simulink model "sistema_completo_con_observador_de_estado"  (R2023b)
settings: Solver=VariableStepAuto  StartTime=0.0  StopTime=10.0  RelTol=1e-3
values from neighbouring files (symbols this model uses):
  alpha_Cu = 3.9e-3    (= 0.0039)    [controlador_foc_simulink.m]    (also in parametros_planta.m; params_subsistema_termico.m; sistema_completo_en_codigo.m)
  ba_num = Jeq_ctrl*n_pid*wn_pid    (= 0.0395694444444)    [controlador_foc_simulink.m]    (also in sistema_completo_en_codigo.m)
  beq_nom = bm + bl_nom/r^2    (= 2.19444444444e-05)    [parametros_planta.m]    (also in params_subsistema_mecanico.m; sistema_completo_en_codigo.m)
  Cts = 0.818    [parametros_planta.m]    (also in params_subsistema_termico.m)
  g = 9.80665    [controlador_foc_simulink.m]    (also in parametros_planta.m; params_subsistema_mecanico.m; sistema_completo_en_codigo.m)
  Jeq_nom = Jm + Jl_nom/r^2    (= 1.97847222222e-05)    [params_subsistema_mecanico.m]    (also in sistema_completo_en_codigo.m)
  kg_eq_nom = g*kl_nom/r    (= 0.0204305208333)    [params_subsistema_mecanico.m]    (also in sistema_completo_en_codigo.m)
  kl_nom = m*Lcm + ml_nom*Ll    (= 0.25)    [controlador_foc_simulink.m]    (also in params_subsistema_mecanico.m; sistema_completo_en_codigo.m)
  Ksa_num = Jeq_ctrl*n_pid*wn_pid^2    (= 31.6555555556)    [controlador_foc_simulink.m]    (also in sistema_completo_en_codigo.m)
  Ksia_num = Jeq_ctrl*wn_pid^3    (= 10129.7777778)    [controlador_foc_simulink.m]    (also in sistema_completo_en_codigo.m)
  L_d = 6.6e-3    (= 0.0066)    [controlador_foc_simulink.m]    (also in params_subsistema_electromagnetico.m; sistema_completo_en_codigo.m)
  L_l = 0.8e-3    (= 0.0008)    [controlador_foc_simulink.m]    (also in params_subsistema_electromagnetico.m; sistema_completo_en_codigo.m)
  L_q = 5.8e-3    (= 0.0058)    [controlador_foc_simulink.m]    (also in params_subsistema_electromagnetico.m; sistema_completo_en_codigo.m)
  lambda_m = 0.016    [controlador_foc_simulink.m]    (also in parametros_planta.m; params_subsistema_electromagnetico.m; sistema_completo_en_codigo.m)
  Pp = 3    [controlador_foc_simulink.m]    (also in parametros_planta.m; params_subsistema_electromagnetico.m; sistema_completo_en_codigo.m)
  r = 120.0    (= 120)    [controlador_foc_simulink.m]    (also in parametros_planta.m; params_subsistema_mecanico.m; sistema_completo_en_codigo.m)
  Rs_REF = 1.02    [controlador_foc_simulink.m]    (also in parametros_planta.m; params_subsistema_termico.m; sistema_completo_en_codigo.m)
  Rts_amb = 146.7    [parametros_planta.m]    (also in params_subsistema_termico.m)
  Tamb = Tamb_max    (= 40)    [parametros_planta.m]    (also in params_subsistema_termico.m; sistema_completo_en_codigo.m)
  Ts_REF = 20.0    (= 20)    [controlador_foc_simulink.m]    (also in parametros_planta.m; params_subsistema_termico.m; sistema_completo_en_codigo.m)
settings Model: Creator=Pc  LastModifiedBy=Pc

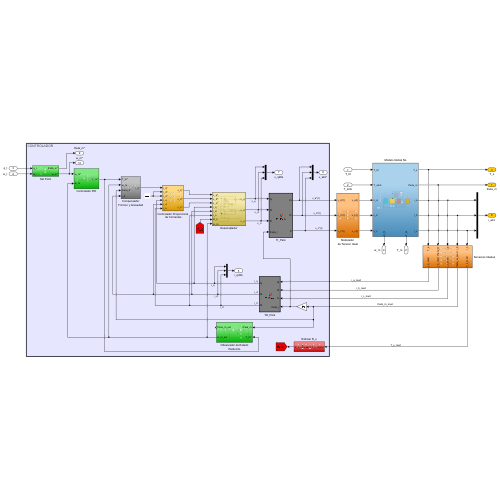
[thumbnail: Simulink's stored preview of the top-level diagram]
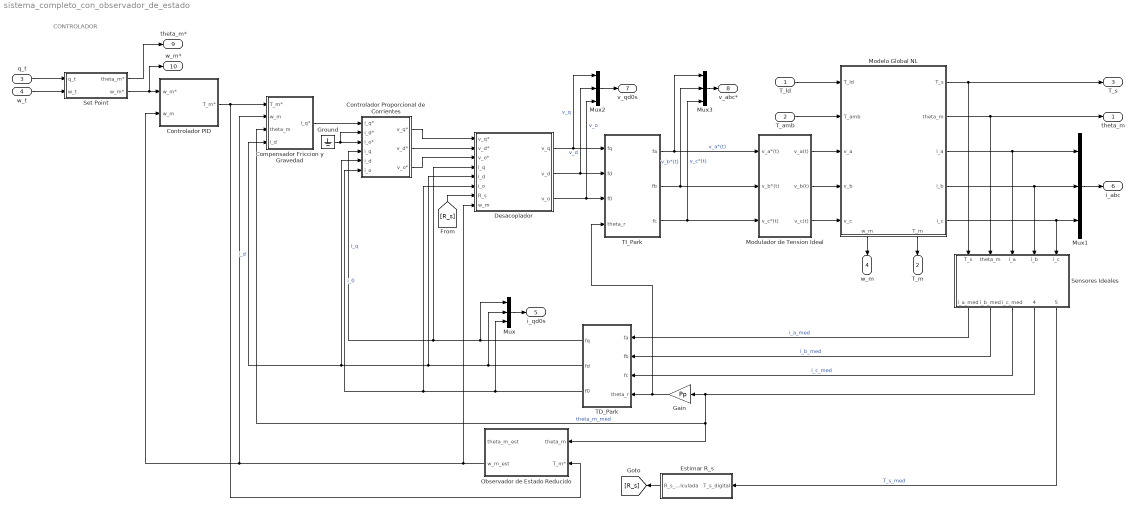
== system sistema_completo_con_observador_de_estado ==
  note: CONTROLADOR
  T_ld : Inport
  T_amb : Inport  Port=2
  q_t : Inport  Port=3
  w_t : Inport  Port=4
  Compensador Friccion y Gravedad : Subsystem
  Controlador PID : Subsystem
  Controlador Proporcional de Corrientes : Subsystem
  Desacoplador : Subsystem
  Estimar R_s : Subsystem
  Gain : Gain  Gain=Pp
  Ground : Ground
  Modelo Global NL : Subsystem
      settings: PortSchema="{\"entries\":[{\"content\":{\"sides\":[{\"content\":{\"connectorIds\":[\"In1\",\"In2\",\"In3\",\"In4\",\"In5\"]},\"type\":\"ConnectorPlacement.EquallySpacedRectSide\",\"uuid\":\"386252be-5f39-4928-a151-52e681895a84\"},{\"content\":{\"connectorIds\":[\"Out1\",\"Out2\",\"Out3\",\"Out4\",\"Out5\"],\"side\":\"RIGHT\"},\"type\":\"ConnectorPlacement.EquallySpacedRectSide\",\"uuid\":\"aee83b90-e95b-4477-b157-a5534e7c5e6c\"},{\"content\":{\"side\":\"TOP\"},\"type\":\"ConnectorPlacement.EquallySpacedRectSide\",\"uuid\":\"e739b3f7-cae1-4498-b396-d13f7405e232\"},{\"content\":{\"connectorIds\":[\"Out6\",\"Out7\"],\"side\":\"BOTTOM\"},\"type\":\"ConnectorPlacement.EquallySpacedRectSide\",\"uuid\":\"86304fed-22cd-46a2-87e5-e7bae1c5cedf\"}]},\"type\":\"ConnectorPlacement.EquallySpacedConnector\",\"uuid\":\"c0eb110b-b212-4702-a1d5-9ec3ac2ff196\"}],\"packageUris\":[\"http://schema.mathworks.com/mf0/Connector/R2020b\"],\"version\":\"1.0\"}"
  Modulador de Tension Ideal : Subsystem
  Mux{,1..3} (4 alike) : Mux  Inputs=3
  Observador de Estado Reducido : Subsystem
  Sensores Ideales : Subsystem
  Set Point : Subsystem
  TD_Park : MATLAB Function  TreatAsAtomicUnit=on
  TI_Park : MATLAB Function  TreatAsAtomicUnit=on
  theta_m : Outport
  T_m : Outport  Port=2
  T_s : Outport  Port=3
  w_m : Outport  Port=4
  i_qd0s : Outport  Port=5
  i_abc : Outport  Port=6
  v_qd0s : Outport  Port=7
  v_abc* : Outport  Port=8
  theta_m* : Outport  Port=9
  w_m* : Outport  Port=10
  wires:
  Sensores Ideales/2(i_b_med) -> TD_Park/2(fb)  "i_b_med"
  Modulador de Tension Ideal/2(v_b(t)) -> Modelo Global NL/4(v_b)
  Mux2/1 -> v_qd0s/1
  TI_Park/2(fb) -> Modulador de Tension Ideal/2(v_b*(t)), Mux3/2  "v_b*(t)"
  Desacoplador/3(v_o) -> Mux2/3, TI_Park/3(f0)  "v_o"
  Mux1/1 -> i_abc/1
  Sensores Ideales/4(theta_m_med) -> Observador de Estado Reducido/1(theta_m), Compensador Friccion y Gravedad/3(theta_m), Gain/1  "theta_m_med"
  TD_Park/2(fd) -> Compensador Friccion y Gravedad/4(i_d), Controlador Proporcional de Corrientes/5(i_d), Desacoplador/5(i_d), Mux/2  "i_d"
  Modelo Global NL/1(T_s) -> T_s/1, Sensores Ideales/1(T_s)
  Modulador de Tension Ideal/1(v_a(t)) -> Modelo Global NL/3(v_a)
  Desacoplador/1(v_q) -> Mux2/1, TI_Park/1(fq)  "v_q"
  TD_Park/1(fq) -> Desacoplador/4(i_q), Controlador Proporcional de Corrientes/4(i_q), Mux/1  "i_q"
  TI_Park/3(fc) -> Modulador de Tension Ideal/3(v_c*(t)), Mux3/3  "v_c*(t)"
  Modelo Global NL/5(i_c) -> Mux1/3, Sensores Ideales/5(i_c)
  Mux/1 -> i_qd0s/1
  Gain/1 -> TI_Park/4(theta_r), TD_Park/4(theta_r)
  Modelo Global NL/7(T_m) -> T_m/1
  Mux3/1 -> v_abc*/1
  Sensores Ideales/3(i_c_med) -> TD_Park/3(fc)  "i_c_med"
  TD_Park/3(f0) -> Controlador Proporcional de Corrientes/6(i_o), Desacoplador/6(i_o), Mux/3  "i_0"
  Sensores Ideales/1(i_a_med) -> TD_Park/1(fa)  "i_a_med"
  Modulador de Tension Ideal/3(v_c(t)) -> Modelo Global NL/5(v_c)
  Modelo Global NL/2(theta_m) -> theta_m/1, Sensores Ideales/2(theta_m)
  T_amb/1 -> Modelo Global NL/2(T_amb)
  T_ld/1 -> Modelo Global NL/1(T_ld)
  TI_Park/1(fa) -> Mux3/1, Modulador de Tension Ideal/1(v_a*(t))  "v_a*(t)"
  Modelo Global NL/3(i_a) -> Mux1/1, Sensores Ideales/3(i_a)
  Modelo Global NL/4(i_b) -> Mux1/2, Sensores Ideales/4(i_b)
  Desacoplador/2(v_d) -> Mux2/2, TI_Park/2(fd)  "v_d"
  Controlador Proporcional de Corrientes/2(v_d*) -> Desacoplador/2(v_d*)
  Controlador Proporcional de Corrientes/3(v_o*) -> Desacoplador/3(v_o*)
  Controlador Proporcional de Corrientes/1(v_q*) -> Desacoplador/1(v_q*)
  Ground/1 -> Controlador Proporcional de Corrientes/2(i_d*), Controlador Proporcional de Corrientes/3(i_o*)
  Compensador Friccion y Gravedad/1(i_q*) -> Controlador Proporcional de Corrientes/1(i_q*)
  Controlador PID/1(T_m*) -> Observador de Estado Reducido/2(T_m*), Compensador Friccion y Gravedad/1(T_m*)
  q_t/1 -> Set Point/1(q_t)
  w_t/1 -> Set Point/2(w_t)
  Set Point/2(w_m*) -> w_m*/1, Controlador PID/1(w_m*)
  Set Point/1(theta_m*) -> theta_m*/1
  Estimar R_s/1(R_s_calculada) -> [R_s]
  [R_s] -> Desacoplador/7(R_s)
  Modelo Global NL/6(w_m) -> w_m/1
  Observador de Estado Reducido/2(w_m_est) -> Controlador PID/2(w_m), Compensador Friccion y Gravedad/2(w_m), Desacoplador/8(w_m)
  Sensores Ideales/5(T_s_med) -> Estimar R_s/1(T_s_digital)  "T_s_med"

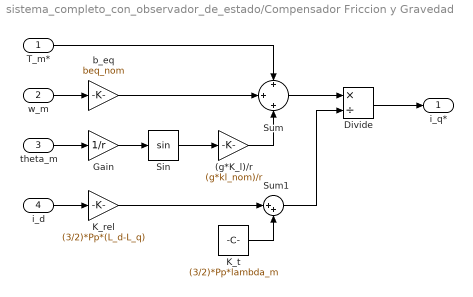
== system sistema_completo_con_observador_de_estado/Compensador Friccion y Gravedad ==
  T_m* : Inport
  w_m : Inport  Port=2
  theta_m : Inport  Port=3
  i_d : Inport  Port=4
  (g*K_l)/r : Gain  Gain=(g*kl_nom)/r
  Divide : Product  Inputs=*/
  Gain : Gain  Gain=1/r
  K_rel : Gain  Gain=(3/2)*Pp*(L_d-L_q)
  K_t : Constant  Value=(3/2)*Pp*lambda_m
  Sin : Trigonometry
  Sum : Sum  Inputs=+|+|+
  Sum1 : Sum  Inputs=|++
  b_eq : Gain  Gain=beq_nom
  i_q* : Outport
  wires:
  i_d/1 -> K_rel/1
  T_m*/1 -> Sum/1
  Sin/1 -> (g*K_l)/r/1
  K_t/1 -> Sum1/2
  (g*K_l)/r/1 -> Sum/3
  Sum1/1 -> Divide/2
  Gain/1 -> Sin/1
  b_eq/1 -> Sum/2
  K_rel/1 -> Sum1/1
  w_m/1 -> b_eq/1
  Sum/1 -> Divide/1
  Divide/1 -> i_q*/1
  theta_m/1 -> Gain/1

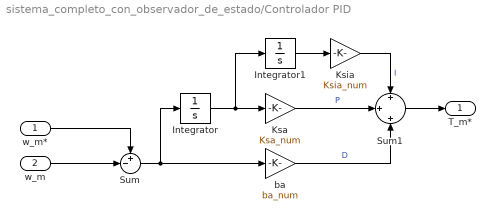
== system sistema_completo_con_observador_de_estado/Controlador PID ==
  w_m* : Inport
  w_m : Inport  Port=2
  Integrator : Integrator
  Integrator1 : Integrator
  Ksa : Gain  Gain=Ksa_num
  Ksia : Gain  Gain=Ksia_num
  Sum : Sum  Inputs=+-|
  Sum1 : Sum  Inputs=+|+|+
  ba : Gain  Gain=ba_num
  T_m* : Outport
  wires:
  Sum1/1 -> T_m*/1
  Ksa/1 -> Sum1/2  "P"
  Ksia/1 -> Sum1/1  "I"
  ba/1 -> Sum1/3  "D"
  Integrator/1 -> Integrator1/1, Ksa/1
  Integrator1/1 -> Ksia/1
  Sum/1 -> Integrator/1, ba/1
  w_m*/1 -> Sum/1
  w_m/1 -> Sum/2

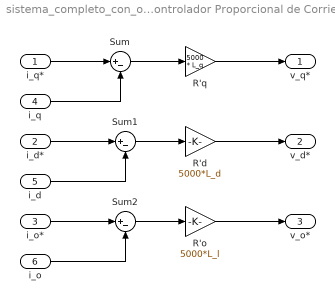
== system sistema_completo_con_observador_de_estado/Controlador Proporcional de Corrientes ==
  i_q* : Inport
  i_d* : Inport  Port=2
  i_o* : Inport  Port=3
  i_q : Inport  Port=4
  i_d : Inport  Port=5
  i_o : Inport  Port=6
  R'd : Gain  Gain=5000*L_d
  R'o : Gain  Gain=5000*L_l
  R'q : Gain  Gain=5000 * L_q
  Sum : Sum  Inputs=|+-
  Sum1 : Sum  Inputs=|+-
  Sum2 : Sum  Inputs=|+-
  v_q* : Outport
  v_d* : Outport  Port=2
  v_o* : Outport  Port=3
  wires:
  R'd/1 -> v_d*/1
  i_q/1 -> Sum/2
  i_d*/1 -> Sum1/1
  R'o/1 -> v_o*/1
  i_o*/1 -> Sum2/1
  Sum/1 -> R'q/1
  Sum1/1 -> R'd/1
  i_o/1 -> Sum2/2
  Sum2/1 -> R'o/1
  R'q/1 -> v_q*/1
  i_d/1 -> Sum1/2
  i_q*/1 -> Sum/1

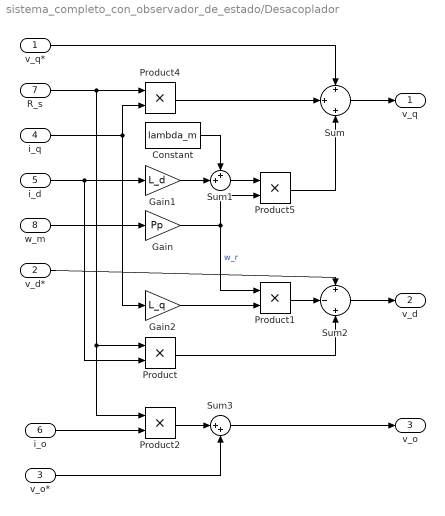
== system sistema_completo_con_observador_de_estado/Desacoplador ==
  v_q* : Inport
  v_d* : Inport  Port=2
  v_o* : Inport  Port=3
  i_q : Inport  Port=4
  i_d : Inport  Port=5
  i_o : Inport  Port=6
  R_s : Inport  Port=7
  w_m : Inport  Port=8
  Constant : Constant  Value=lambda_m
  Gain : Gain  Gain=Pp
  Gain1 : Gain  Gain=L_d
  Gain2 : Gain  Gain=L_q
  Product{,1..2,4..5} (5 alike) : Product
  Sum : Sum  Inputs=+|+|+
  Sum1 : Sum  Inputs=++|
  Sum2 : Sum  Inputs=+|-|+
  Sum3 : Sum  Inputs=|++
  v_q : Outport
  v_d : Outport  Port=2
  v_o : Outport  Port=3
  wires:
  R_s/1 -> Product/1, Product2/1, Product4/1
  Product2/1 -> Sum3/1
  v_d*/1 -> Sum2/1
  Gain/1 -> Product1/1, Product5/2  "w_r"
  Gain1/1 -> Sum1/2
  Product/1 -> Sum2/3
  Sum3/1 -> v_o/1
  i_d/1 -> Gain1/1, Product/2
  Product5/1 -> Sum/3
  Product1/1 -> Sum2/2
  Product4/1 -> Sum/2
  v_q*/1 -> Sum/1
  i_q/1 -> Gain2/1, Product4/2
  Sum/1 -> v_q/1
  i_o/1 -> Product2/2
  Sum1/1 -> Product5/1
  Sum2/1 -> v_d/1
  v_o*/1 -> Sum3/2
  w_m/1 -> Gain/1
  Constant/1 -> Sum1/1
  Gain2/1 -> Product1/2

== system sistema_completo_con_observador_de_estado/Estimar R_s ==
  T_s_digital : Inport
  Constant3 : Constant
  Rs_ref : Gain  Gain=Rs_REF
  Sum3 : Sum  Inputs=|+-
  Sum4 : Sum  Inputs=|++
  Ts_ref : Constant  Value=Ts_REF
  alpha_Cu : Gain  Gain=alpha_Cu
  R_s_calculada : Outport
  wires:
  Ts_ref/1 -> Sum3/2
  T_s_digital/1 -> Sum3/1
  Constant3/1 -> Sum4/2
  Rs_ref/1 -> R_s_calculada/1  "R_s"
  Sum4/1 -> Rs_ref/1
  Sum3/1 -> alpha_Cu/1
  alpha_Cu/1 -> Sum4/1

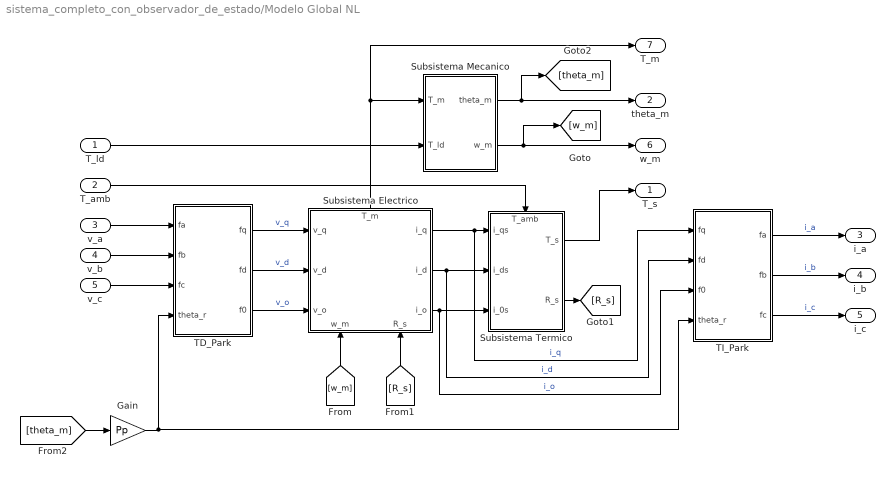
== system sistema_completo_con_observador_de_estado/Modelo Global NL ==
  T_ld : Inport
  T_amb : Inport  Port=2
  v_a : Inport  Port=3
  v_b : Inport  Port=4
  v_c : Inport  Port=5
  Gain : Gain  Gain=Pp
  Subsistema Electrico : Subsystem
      settings: PortSchema="{\"entries\":[{\"content\":{\"sides\":[{\"content\":{\"connectorIds\":[\"In1\",\"In2\",\"In3\"]},\"type\":\"ConnectorPlacement.EquallySpacedRectSide\",\"uuid\":\"c7eb63ae-4015-4be9-a2f8-5ddbad38e871\"},{\"content\":{\"connectorIds\":[\"Out1\",\"Out2\",\"Out3\"],\"side\":\"RIGHT\"},\"type\":\"ConnectorPlacement.EquallySpacedRectSide\",\"uuid\":\"ed205027-9864-417a-9d2b-6eeb723ffec2\"},{\"content\":{\"connectorIds\":[\"Out4\"],\"side\":\"TOP\"},\"type\":\"ConnectorPlacement.EquallySpacedRectSide\",\"uuid\":\"5c5dee03-5728-4212-8fc2-a453d3484329\"},{\"content\":{\"connectorIds\":[\"In4\",\"In5\"],\"side\":\"BOTTOM\"},\"type\":\"ConnectorPlacement.EquallySpacedRectSide\",\"uuid\":\"494df340-b6d5-4f09-932e-9dbff39af1cf\"}]},\"type\":\"ConnectorPlacement.EquallySpacedConnector\",\"uuid\":\"0eeaea4c-3d80-4ebb-8c27-59b1b18764e9\"}],\"packageUris\":[\"http://schema.mathworks.com/mf0/Connector/R2020b\"],\"version\":\"1.0\"}"
  Subsistema Mecanico : Subsystem
  Subsistema Termico : Subsystem
      settings: PortSchema="{\"entries\":[{\"content\":{\"sides\":[{\"content\":{\"connectorIds\":[\"In1\",\"In2\",\"In3\"]},\"type\":\"ConnectorPlacement.EquallySpacedRectSide\",\"uuid\":\"5b1848a7-84bd-4673-a3fa-3976b4d0d5b9\"},{\"content\":{\"connectorIds\":[\"Out1\",\"Out2\"],\"side\":\"RIGHT\"},\"type\":\"ConnectorPlacement.EquallySpacedRectSide\",\"uuid\":\"feff3f8a-cd7c-43b1-91c3-7ab01b0b33a6\"},{\"content\":{\"connectorIds\":[\"In4\"],\"side\":\"TOP\"},\"type\":\"ConnectorPlacement.EquallySpacedRectSide\",\"uuid\":\"8de0b1b6-142f-442a-a92f-2baa615c6322\"}]},\"type\":\"ConnectorPlacement.EquallySpacedConnector\",\"uuid\":\"046fcb24-e0d9-4784-a784-7e36f9acbfbc\"}],\"packageUris\":[\"http://schema.mathworks.com/mf0/Connector/R2020b\"],\"version\":\"1.0\"}"
  TD_Park : MATLAB Function  TreatAsAtomicUnit=on
  TI_Park : MATLAB Function  TreatAsAtomicUnit=on
  T_s : Outport
  theta_m : Outport  Port=2
  i_a : Outport  Port=3
  i_b : Outport  Port=4
  i_c : Outport  Port=5
  w_m : Outport  Port=6
  T_m : Outport  Port=7
  wires:
  Subsistema Mecanico/1(theta_m) -> theta_m/1, [theta_m]
  TD_Park/2(fd) -> Subsistema Electrico/2(v_d)  "v_d"
  Subsistema Termico/1(T_s) -> T_s/1
  TD_Park/3(f0) -> Subsistema Electrico/3(v_o)  "v_o"
  Subsistema Mecanico/2(w_m) -> w_m/1, [w_m]
  [R_s] -> Subsistema Electrico/5(R_s)
  TI_Park/1(fa) -> i_a/1  "i_a"
  TD_Park/1(fq) -> Subsistema Electrico/1(v_q)  "v_q"
  Subsistema Electrico/4(T_m) -> T_m/1, Subsistema Mecanico/1(T_m)
  v_c/1 -> TD_Park/3(fc)
  Subsistema Electrico/2(i_d) -> Subsistema Termico/2(i_ds), TI_Park/2(fd)  "i_d"
  Subsistema Termico/2(R_s) -> [R_s]
  T_amb/1 -> Subsistema Termico/4(T_amb)
  T_ld/1 -> Subsistema Mecanico/2(T_ld)
  Subsistema Electrico/3(i_o) -> Subsistema Termico/3(i_0s), TI_Park/3(f0)  "i_o"
  TI_Park/2(fb) -> i_b/1  "i_b"
  Subsistema Electrico/1(i_q) -> TI_Park/1(fq), Subsistema Termico/1(i_qs)  "i_q"
  v_a/1 -> TD_Park/1(fa)
  v_b/1 -> TD_Park/2(fb)
  [w_m] -> Subsistema Electrico/4(w_m)
  TI_Park/3(fc) -> i_c/1  "i_c"
  [theta_m] -> Gain/1
  Gain/1 -> TD_Park/4(theta_r), TI_Park/4(theta_r)

== system sistema_completo_con_observador_de_estado/Modulador de Tension Ideal ==
  v_a*(t) : Inport
  v_b*(t) : Inport  Port=2
  v_c*(t) : Inport  Port=3
  Gain : Gain
  Gain1 : Gain
  Gain2 : Gain
  v_a(t) : Outport
  v_b(t) : Outport  Port=2
  v_c(t) : Outport  Port=3
  wires:
  v_a*(t)/1 -> Gain/1
  Gain/1 -> v_a(t)/1
  v_b*(t)/1 -> Gain1/1
  Gain1/1 -> v_b(t)/1
  v_c*(t)/1 -> Gain2/1
  Gain2/1 -> v_c(t)/1

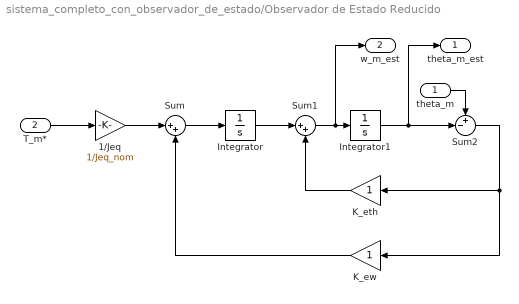
== system sistema_completo_con_observador_de_estado/Observador de Estado Reducido ==
  theta_m : Inport
  T_m* : Inport  Port=2
  1/Jeq : Gain  Gain=1/Jeq_nom
  Integrator : Integrator
  Integrator1 : Integrator
  K_eth : Gain
  K_ew : Gain
  Sum : Sum  Inputs=|++
  Sum1 : Sum  Inputs=|++
  Sum2 : Sum  Inputs=+-|
  theta_m_est : Outport
  w_m_est : Outport  Port=2
  wires:
  Integrator1/1 -> theta_m_est/1, Sum2/2
  Sum2/1 -> K_eth/1, K_ew/1
  Sum1/1 -> w_m_est/1, Integrator1/1
  theta_m/1 -> Sum2/1
  K_eth/1 -> Sum1/2
  Sum/1 -> Integrator/1
  1/Jeq/1 -> Sum/1
  K_ew/1 -> Sum/2
  T_m*/1 -> 1/Jeq/1
  Integrator/1 -> Sum1/1

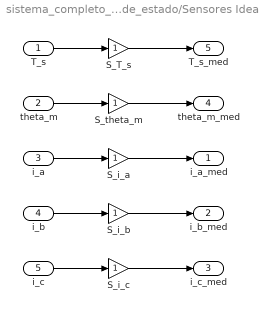
== system sistema_completo_con_observador_de_estado/Sensores Ideales ==
  T_s : Inport
  theta_m : Inport  Port=2
  i_a : Inport  Port=3
  i_b : Inport  Port=4
  i_c : Inport  Port=5
  S_T_s : Gain
  S_i_a : Gain
  S_i_b : Gain
  S_i_c : Gain
  S_theta_m : Gain
  i_a_med : Outport
  i_b_med : Outport  Port=2
  i_c_med : Outport  Port=3
  theta_m_med : Outport  Port=4
  T_s_med : Outport  Port=5
  wires:
  i_a/1 -> S_i_a/1
  T_s/1 -> S_T_s/1
  S_theta_m/1 -> theta_m_med/1
  theta_m/1 -> S_theta_m/1
  S_i_c/1 -> i_c_med/1
  i_b/1 -> S_i_b/1
  i_c/1 -> S_i_c/1
  S_T_s/1 -> T_s_med/1
  S_i_b/1 -> i_b_med/1
  S_i_a/1 -> i_a_med/1

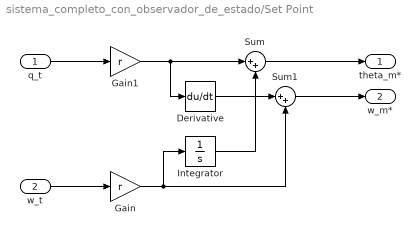
== system sistema_completo_con_observador_de_estado/Set Point ==
  q_t : Inport
  w_t : Inport  Port=2
  Derivative : Derivative
  Gain : Gain  Gain=r
  Gain1 : Gain  Gain=r
  Integrator : Integrator
  Sum : Sum  Inputs=|++
  Sum1 : Sum  Inputs=|++
  theta_m* : Outport
  w_m* : Outport  Port=2
  wires:
  Gain1/1 -> Derivative/1, Sum/1
  Derivative/1 -> Sum1/1
  Gain/1 -> Integrator/1, Sum1/2
  Integrator/1 -> Sum/2
  Sum/1 -> theta_m*/1
  Sum1/1 -> w_m*/1
  w_t/1 -> Gain/1
  q_t/1 -> Gain1/1

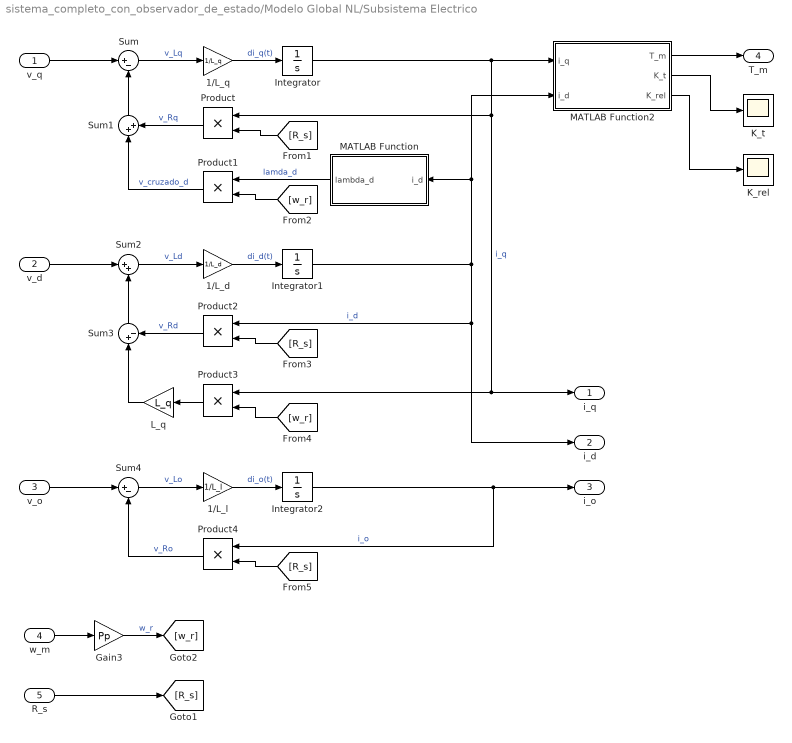
== system sistema_completo_con_observador_de_estado/Modelo Global NL/Subsistema Electrico ==
  v_q : Inport
  v_d : Inport  Port=2
  v_o : Inport  Port=3
  w_m : Inport  Port=4
  R_s : Inport  Port=5
  1/L_d : Gain  Gain=1/L_d
  1/L_l : Gain  Gain=1/L_l
  1/L_q : Gain  Gain=1/L_q
  Gain3 : Gain  Gain=Pp
  Integrator : Integrator
  Integrator1 : Integrator
  Integrator2 : Integrator
  K_rel : Scope
  K_t : Scope
  L_q : Gain  Gain=L_q
  MATLAB Function : MATLAB Function  TreatAsAtomicUnit=on
  MATLAB Function2 : MATLAB Function  TreatAsAtomicUnit=on
  Product{,1..4} (5 alike) : Product
  Sum : Sum  Inputs=|+-
  Sum1 : Sum  Inputs=|++
  Sum2 : Sum  Inputs=|++
  Sum3 : Sum  Inputs=|+-
  Sum4 : Sum  Inputs=|+-
  i_q : Outport
  i_d : Outport  Port=2
  i_o : Outport  Port=3
  T_m : Outport  Port=4
  wires:
  Integrator/1 -> MATLAB Function2/1(i_q), Product/1, i_q/1, Product3/1  "i_q"
  Sum3/1 -> Sum2/2
  Product1/1 -> Sum1/1  "v_cruzado_d"
  Integrator1/1 -> MATLAB Function2/2(i_d), MATLAB Function/1(i_d), i_d/1, Product2/1  "i_d"
  Sum1/1 -> Sum/2
  1/L_d/1 -> Integrator1/1  "di_d(t)"
  MATLAB Function/1(lambda_d) -> Product1/1  "lamda_d"
  Sum4/1 -> 1/L_l/1  "v_Lo"
  [w_r] -> Product3/2
  Sum/1 -> 1/L_q/1  "v_Lq"
  1/L_l/1 -> Integrator2/1  "di_o(t)"
  Integrator2/1 -> i_o/1, Product4/1  "i_o"
  Product2/1 -> Sum3/2  "v_Rd"
  Product/1 -> Sum1/2  "v_Rq"
  [R_s] -> Product4/2
  Product3/1 -> L_q/1
  1/L_q/1 -> Integrator/1  "di_q(t)"
  Sum2/1 -> 1/L_d/1  "v_Ld"
  v_q/1 -> Sum/1
  [R_s] -> Product/2
  Product4/1 -> Sum4/2  "v_Ro"
  [w_r] -> Product1/2
  [R_s] -> Product2/2
  L_q/1 -> Sum3/1
  v_d/1 -> Sum2/1
  v_o/1 -> Sum4/1
  MATLAB Function2/1(T_m) -> T_m/1
  MATLAB Function2/3(K_rel) -> K_rel/1
  MATLAB Function2/2(K_t) -> K_t/1
  w_m/1 -> Gain3/1
  R_s/1 -> [R_s]
  Gain3/1 -> [w_r]  "w_r"

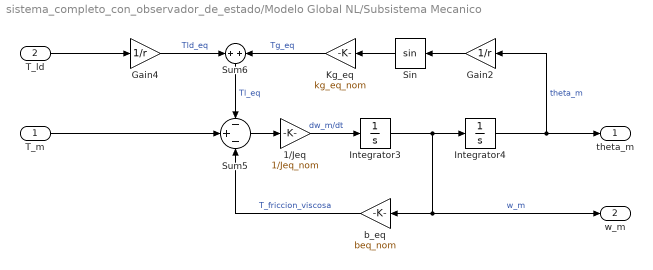
== system sistema_completo_con_observador_de_estado/Modelo Global NL/Subsistema Mecanico ==
  T_m : Inport
  T_ld : Inport  Port=2
  1/Jeq : Gain  Gain=1/Jeq_nom
  Gain2 : Gain  Gain=1/r
  Gain4 : Gain  Gain=1/r
  Integrator3 : Integrator
  Integrator4 : Integrator
  Kg_eq : Gain  Gain=kg_eq_nom
  Sin : Trigonometry
  Sum5 : Sum  Inputs=-+-
  Sum6 : Sum  Inputs=+|+
  b_eq : Gain  Gain=beq_nom
  theta_m : Outport
  w_m : Outport  Port=2
  wires:
  Sin/1 -> Kg_eq/1
  Gain4/1 -> Sum6/1  "Tld_eq"
  Integrator4/1 -> theta_m/1, Gain2/1  "theta_m"
  Kg_eq/1 -> Sum6/2  "Tg_eq"
  Sum5/1 -> 1/Jeq/1
  b_eq/1 -> Sum5/3  "T_friccion_viscosa"
  T_m/1 -> Sum5/2
  Gain2/1 -> Sin/1
  Sum6/1 -> Sum5/1  "Tl_eq"
  Integrator3/1 -> w_m/1, b_eq/1, Integrator4/1  "w_m"
  T_ld/1 -> Gain4/1
  1/Jeq/1 -> Integrator3/1  "dw_m/dt"

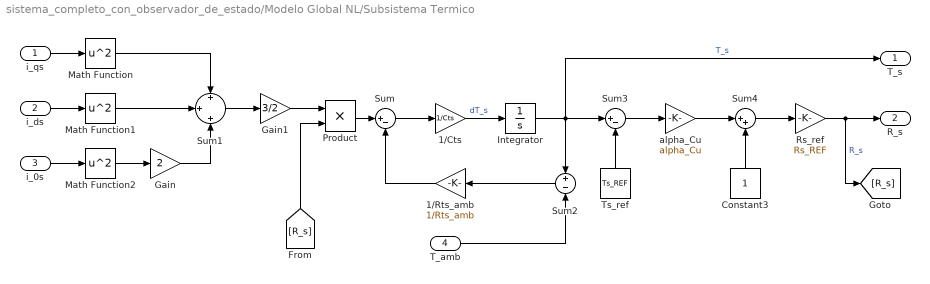
== system sistema_completo_con_observador_de_estado/Modelo Global NL/Subsistema Termico ==
  i_qs : Inport
  i_ds : Inport  Port=2
  i_0s : Inport  Port=3
  T_amb : Inport  Port=4
  1/Cts : Gain  Gain=1/Cts
  1/Rts_amb : Gain  Gain=1/Rts_amb
  Constant3 : Constant
  Gain : Gain  Gain=2
  Gain1 : Gain  Gain=3/2
  Integrator : Integrator  InitialCondition=Tamb
  Math Function : Math  Operator=square
  Math Function1 : Math  Operator=square
  Math Function2 : Math  Operator=square
  Product : Product
  Rs_ref : Gain  Gain=Rs_REF
  Sum : Sum  Inputs=|+-
  Sum1 : Sum  Inputs=+|+|+
  Sum2 : Sum  Inputs=+-
  Sum3 : Sum  Inputs=|+-
  Sum4 : Sum  Inputs=|++
  Ts_ref : Constant  Value=Ts_REF
  alpha_Cu : Gain  Gain=alpha_Cu
  T_s : Outport
  R_s : Outport  Port=2
  wires:
  1/Cts/1 -> Integrator/1  "dT_s"
  Sum3/1 -> alpha_Cu/1
  Rs_ref/1 -> R_s/1, [R_s]  "R_s"
  Sum4/1 -> Rs_ref/1
  [R_s] -> Product/2
  i_ds/1 -> Math Function1/1
  Constant3/1 -> Sum4/2
  Integrator/1 -> T_s/1, Sum2/1, Sum3/1  "T_s"
  Math Function1/1 -> Sum1/2
  alpha_Cu/1 -> Sum4/1
  Sum2/1 -> 1/Rts_amb/1
  Product/1 -> Sum/1
  i_qs/1 -> Math Function/1
  Sum/1 -> 1/Cts/1
  T_amb/1 -> Sum2/2
  Math Function/1 -> Sum1/1
  i_0s/1 -> Math Function2/1
  1/Rts_amb/1 -> Sum/2
  Ts_ref/1 -> Sum3/2
  Math Function2/1 -> Gain/1
  Gain/1 -> Sum1/3
  Sum1/1 -> Gain1/1
  Gain1/1 -> Product/1

== matlab function sistema_completo_con_observador_de_estado/TD_Park ==
  data: fa input; fq output; fb input; fc input; theta_r input; fd output; f0 output
function [fq, fd, f0] = T_Park(fa, fb, fc, theta_r)
%#codegen
% Transformada directa de Park: abc -> qd0
% Convención usada:
% fq: eje q
% fd: eje d
% f0: componente homopolar

c1 = cos(theta_r);
c2 = cos(theta_r - 2*pi/3);
c3 = cos(theta_r + 2*pi/3);

s1 = sin(theta_r);
s2 = sin(theta_r - 2*pi/3);
s3 = sin(theta_r + 2*pi/3);

fq = (2/3)*(c1*fa + c2*fb + c3*fc);
fd = (2/3)*(s1*fa + s2*fb + s3*fc);
f0 = (1/3)*(fa + fb + fc);
end

== matlab function sistema_completo_con_observador_de_estado/TI_Park ==
  data: fq input; fa output; fd input; f0 input; theta_r input; fb output; fc output
function [fa, fb, fc] = TI_Park(fq, fd, f0, theta_r)
%#codegen
% Transformada inversa de Park: qd0 -> abc

fa = cos(theta_r)*fq ...
   + sin(theta_r)*fd ...
   + f0;

fb = cos(theta_r - 2*pi/3)*fq ...
   + sin(theta_r - 2*pi/3)*fd ...
   + f0;

fc = cos(theta_r + 2*pi/3)*fq ...
   + sin(theta_r + 2*pi/3)*fd ...
   + f0;
end

== matlab function sistema_completo_con_observador_de_estado/Modelo Global NL/Subsistema Electrico/MATLAB Function ==
  data: i_d input; lambda_d output; lambda_m parameter; L_d parameter
function lambda_d = calcular_flujo_d(i_d, lambda_m, L_d)
    % CALCULAR_FLUJO_D Calcula el flujo magnético total concatenado en el eje directo (d).
    %
    % Entradas:
    %   i_d      : Corriente instantánea en el eje d (Señal dinámica de entrada).
    %   lambda_m : Flujo de los imanes permanentes (Parámetro estático).
    %   L_d      : Inductancia del estator en el eje d (Parámetro estático).
    %
    % Salida:
    %   lambda_d : Flujo magnético total en el eje d.

    % Cálculo: Flujo de imanes + Flujo de reacción del inducido
    lambda_d = lambda_m + L_d * i_d;
end

== matlab function sistema_completo_con_observador_de_estado/Modelo Global NL/Subsistema Electrico/MATLAB Function2 ==
  data: i_q input; i_d input; T_m output; Pp parameter; lambda_m parameter; L_d parameter; L_q parameter; K_t output; K_rel output
function [T_m, K_t, K_rel] = calcular_torque(i_q, i_d, Pp, lambda_m, L_d, L_q)
    % CALCULAR_TORQUE Calcula el torque electromagnético total de la máquina PMSM
    % y sus constantes equivalentes.
    % 
    % Entradas dinámicas (Inports):
    %   i_q      : Corriente en el eje en cuadratura [A].
    %   i_d      : Corriente en el eje directo [A].
    %
    % Parámetros estáticos (Parameters):
    %   P_p      : Número de pares de polos.
    %   lambda_m : Flujo magnético de los imanes permanentes [Wb].
    %   L_d      : Inductancia del eje d [H].
    %   L_q      : Inductancia del eje q [H].
    %
    % Salidas:
    %   T_m      : Torque electromagnético generado [N.m].
    %   K_t      : Constante de torque de alineación [N.m/A].
    %   K_rel    : Constante de torque de reluctancia [N.m/A^2].

    % 1. Cálculo de las constantes 
    K_t = (3/2) * Pp * lambda_m;
    K_rel = (3/2) * Pp * (L_d - L_q);

    % 2. Cálculo del torque electromagnético total
    T_m = K_t * i_q + K_rel * i_d * i_q;
end

== matlab function sistema_completo_con_observador_de_estado/Modelo Global NL/TD_Park ==
  data: fa input; fq output; fb input; fc input; theta_r input; fd output; f0 output
function [fq, fd, f0] = T_Park(fa, fb, fc, theta_r)
%#codegen
% Transformada directa de Park: abc -> qd0
% Convención usada:
% fq: eje q
% fd: eje d
% f0: componente homopolar

c1 = cos(theta_r);
c2 = cos(theta_r - 2*pi/3);
c3 = cos(theta_r + 2*pi/3);

s1 = sin(theta_r);
s2 = sin(theta_r - 2*pi/3);
s3 = sin(theta_r + 2*pi/3);

fq = (2/3)*(c1*fa + c2*fb + c3*fc);
fd = (2/3)*(s1*fa + s2*fb + s3*fc);
f0 = (1/3)*(fa + fb + fc);
end

== matlab function sistema_completo_con_observador_de_estado/Modelo Global NL/TI_Park ==
  data: fq input; fa output; fd input; f0 input; theta_r input; fb output; fc output
function [fa, fb, fc] = TI_Park(fq, fd, f0, theta_r)
%#codegen
% Transformada inversa de Park: qd0 -> abc

fa = cos(theta_r)*fq ...
   + sin(theta_r)*fd ...
   + f0;

fb = cos(theta_r - 2*pi/3)*fq ...
   + sin(theta_r - 2*pi/3)*fd ...
   + f0;

fc = cos(theta_r + 2*pi/3)*fq ...
   + sin(theta_r + 2*pi/3)*fd ...
   + f0;
end
